simulink model "PESO_2021_1"  (R2020b)
settings: Solver=VariableStepAuto  StartTime=0.0  StopTime=20  FixedStep=1e-4  MaxStep=1e-3  RelTol=1e-9
settings Model: Creator=Amir  LastModifiedBy=Amir
settings DataIOCC: ReturnWorkspaceOutputs=off

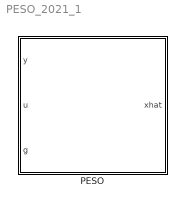
== system PESO_2021_1 ==
  PESO : Subsystem  mask{n=4, tau=10, b=-[5;10;10;5;1], alpha=0.002, x0=10*[1;1;1;1], epsilon_t=1}
      mask prompts: n "Dimension of the system (n):"; tau "Convergence time (tau):"; b "Vector of observer gains (b):"; alpha "Mapping gain (alpha):"; x0 "Initial Estimated state (x0):"; epsilon_t "Switching tolerance (epsilon_t):"
      mask DialogControl DescGroupVar Prompt: Main
      mask DialogControl DescTextVar Prompt: Prescribed-time observer for unknown systems.

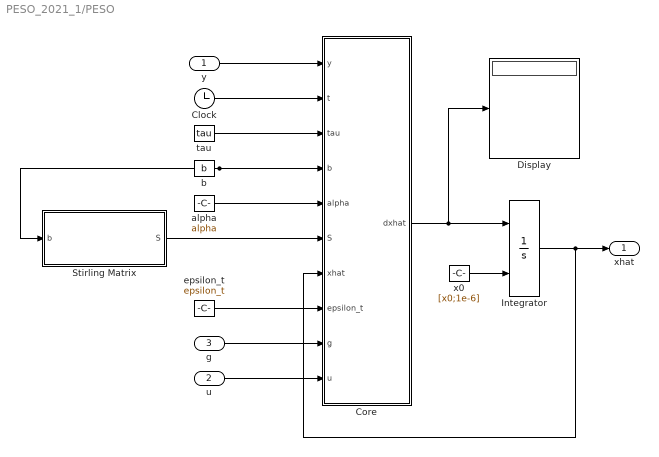
== system PESO_2021_1/PESO ==
  y : Inport
  u : Inport  Port=2
  g : Inport  Port=3
  Clock : Clock
  Core : MATLAB Function  TreatAsAtomicUnit=on
  Display : Display
  Integrator : Integrator  InitialConditionSource=external
  Stirling Matrix : MATLAB Function  TreatAsAtomicUnit=on
  alpha : Constant  Value=alpha
  b : Constant  Value=b
  epsilon_t : Constant  Value=epsilon_t
  tau : Constant  Value=tau
  x0 : Constant  Value=[x0;1e-6]
  xhat : Outport
  wires:
  alpha/1 -> Core/5(alpha)
  b/1 -> Core/4(b), Stirling Matrix/1(b)
  y/1 -> Core/1(y)
  tau/1 -> Core/3(tau)
  Clock/1 -> Core/2(t)
  Stirling Matrix/1(S) -> Core/6(S)
  Core/1(dxhat) -> Display/1, Integrator/1
  x0/1 -> Integrator/2
  Integrator/1 -> xhat/1, Core/7(xhat)
  epsilon_t/1 -> Core/8(epsilon_t)
  u/1 -> Core/10(u)
  g/1 -> Core/9(g)

== matlab function PESO_2021_1/PESO/Core ==
  data: y input size=[1 1]; dxhat output size=[n+1 1]; t input size=[1 1]; tau input size=[1 1]; b input size=[n+1 1]; alpha input size=[1 1]; S input size=[n+2 n+2]; xhat input size=[n+1,1]; epsilon_t input; g input; u input
function dxhat = PTC_gen(y,t,tau,b,alpha,S,xhat,epsilon_t,g,u)

if t>tau-epsilon_t
    
    t=tau-epsilon_t;
    
end

n=length(b)-1;

dxhat=zeros(n+1,1);

p=zeros(n+1,1);

for i=1:n+1
    
    sum=0;
    
    for j=i:n+1
        
        sum=sum+S(j,i)*(b(n-j+2))*(-1)^(j-i)/(alpha^(n-j+2)*(tau-t)^(n-i+2));
        
    end
    
    p(n-i+2)=-S(n+2,i)*(-1)^(n-i+2)/(tau-t)^(n-i+2)+sum;
    
end

for i=1:n-1
    
    dxhat(i)=xhat(i+1)+p(i)*(xhat(1)-y);
    
end

dxhat(n)=xhat(n+1)+p(n)*(xhat(1)-y)+g*u;

dxhat(n+1)=p(n+1)*(xhat(1)-y);

== matlab function PESO_2021_1/PESO/Stirling Matrix ==
  data: b input size=[n+1 1]; S output size=[n+2 n+2]
function S = Stirling_gen(b)

n=length(b)+1;

S=zeros(n,n);

for i=1:n
    
    for j=1:n
        
        if i>=j
            
            m=0;

            for l=0:j-1
    
                sum=1/factorial(j-1)*(-1)^l*(factorial(j-1)/(factorial(l)*factorial(j-1-l)))*(j-1-l)^(i-1);
                
                m=m+sum;
                
            end
            
            S(i,j)=m;
            
        end
        
    end
    
end
